simulink model "SubmarineFault"  (R2019a)
settings: Solver=ode1  StartTime=0.0  StopTime=2.5  FixedStep=Ts_Power  RelTol=1e-3
PostLoadFcn:
  | %% Init for wind PnO models - global system parameters
  | OVERRIDE_SSN_MEMORY_LIMIT=1;
  | Ts=50e-6;
  | % Ts=50e-10;
  | Ts_Power=Ts;
  | Ts_Control=2*Ts;
  | freq = 50;
  | Fnom=freq;
  | Vac=400e3;
InitFcn:
  | %% Init for wind PnO models - global system parameters
  | OVERRIDE_SSN_MEMORY_LIMIT=1;
  | Ts=50e-6;
  | % Ts=50e-10;
  | Ts_Power=Ts;
  | Ts_Control=2*Ts;
  | freq = 50;
  | Fnom=freq;
  | Vac=225e3;
values from neighbouring files (symbols this model uses):
  sub_posCap = 0.16e-006    (= 1.6e-07)    [variable.m]
  sub_posInd = 0.001400563    [variable.m]
  sub_posR = 0.036    [variable.m]
  sub_zeroCap = 0.053333e-006    (= 5.3333e-08)    [variable.m]
  sub_zeroInd = 0.00420169    [variable.m]
  sub_zeroR = 0.108    [variable.m]
  transfo_L1 = 0.05999374    [variable.m]
  transfo_L2 = 0.05999374    [variable.m]
  transfo_R1 = 0.000866667    [variable.m]
  transfo_R2 = 0.00086667    [variable.m]
undefined symbols (not defined in the file or in its folder): D1, D11, Delta, den, DiscIntNeverNeededParam, dx, find_system, gcbh, num, out_Buses, out_WindFarms, sps_rtmsupport
libraries: powerlib x168, simulink x80, powerlib_meascontrol x80, elements x52, eeSinusoidalMeasurement x46, simulink_extras x40, spsVIMeasurementModel x36, eePowerMeasurement x15
(part 6 of 22)

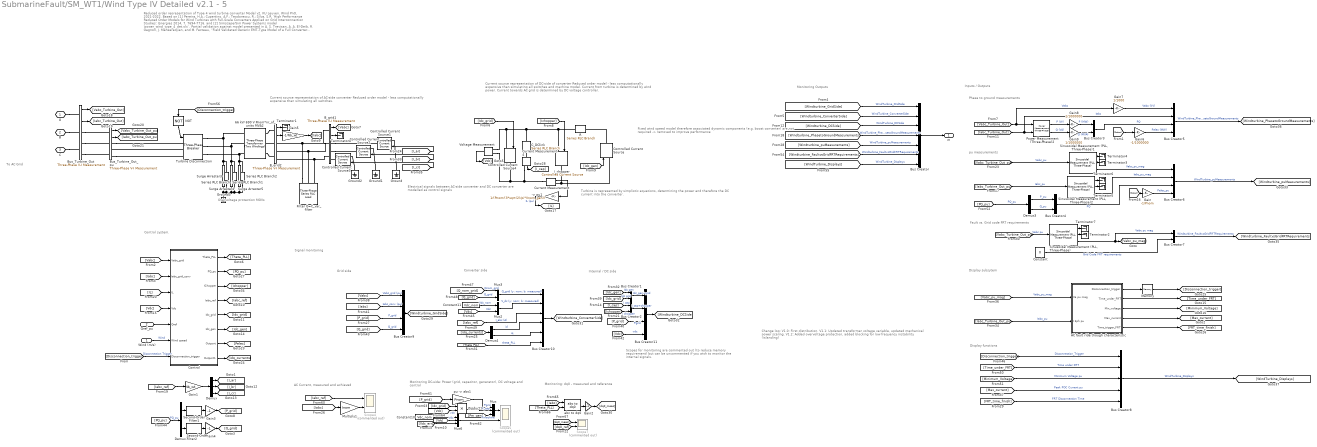
== system SubmarineFault/SM_WT1/Wind Type IV Detailed v2.1 - 5 ==
  note: Fault vs. Grid
      | code FRT
      | requirements
  note: pu measurements
  note: Control system.
  note: AC Current, measured and achieved
  note: Converter side
  note: Monitoring: dq0 - measured and reference
  note: Change log:
      | V1.0: First distribution.
      | V1.1: Updated transformer voltage variable, updated mechanical power scaling.
      | V1.2: Added overvoltage protection, added blocking for low frequency instability (islanding)
  note: Grid side
  note: Overvoltage
      | protection MOVs
  note: Internal / DC side
  note: Fixed wind speed model therefore associated dynamic components (e.g. boost converter) are not required -> removed to improve performance
  note: Scopes for monitoring are commented out (to reduce memory requirement) but can be uncommented if you wish to monitor the internal signals.
  note: Electrical signals between AC-side converter and DC converter are modelled as control signals
  note: Monitoring DC-side: Power (grid, capacitor, generator), DC voltage and control
  note: To AC Grid
  note: Monitoring Outputs
  note: Signal monitoring
  note: Current source representation of AC-side converter
      | Reduced order model - less computationally expensive than simulating all switches.
  note: Turbine is represented by simplistic equations, determining the power and therefore the DC current into the converter.
  note: Current source representation of DC-side of converter
      | Reduced order model - less computationally expensive than simulating all switches and machine model. Current from turbine is determined by wind power. Current towards AC grid is determined by DC voltage controller.
  note: Reduced order representation of Type 4 wind turbine converter
      | Model v2, KU Leuven, Wind PnO, 2021-2022.
      | Based on [1] Pereira, H.A.; Cupertino, A.F.; Teodorescu, R.; Silva, S.R. 'High Performance Reduced Order Models for Wind Turbines with Full-Scale Converters Applied on Grid Interconnection Studies'. Energies 2014, 7, 7694-7716. and [2] Simscape/Sim Power Systems model 'power_wind_type_4_det.slx' . Partial validation against model presented in A. S. Trevisan, A. A. El-Deib, R. Gagnon, J. Mahseredjian, and M. Fecteau, “Field Validated Generic EMT-Type Model of a Full Converter Wind Turbine Based on a Gearless Externally Excited Synchronous Generator,” IEEE Trans. Power Deliv., 2018. Developed with reduced complexity to allow for real time simulation in future sessions.
  note: Phase to ground measurements
  note: Display subsytem
  note: Display functions
  note: Inputs / Outputs
  "Wind (m/s) " : Inport
  Qref_pu : Inport  Port=2
  -> pu1 : Gain  Gain=1/(Pnom/(3*sqrt(2)/pi*Vnom_gen))  SaturateOnIntegerOverflow=on  OutDataTypeStr=Inherit: Same as input  ParamDataTypeStr=Inherit: Same as input
  66 kV/ 690 V Pnom*nr_of_units MVA2 : powerlib/Elements/Three-Phase Transformer (Two Windings)  Winding1Connection=Delta (D11)  Winding2Connection=Yg  CoreType=Three single-phase transformers  SetSaturation=off  Hysteresis=off  DataFile='hysteresis'  SetInitialFlux=off  Measurements=None  UNITS=pu  NominalPower="[Pnom*Nb_wt  freq]"  Winding1=[Vgrid 0.00083333 0.025]  Winding2=[690 0.00083333 0.025]  Rm=500  Lm=Inf  L0=0.5  Saturation=[0 0;0.0024 1.2;1 1.52]  InitialFluxes=[ 0.8 , -0.8 , 0.7 ]  BreakLoop=off  DiscreteSolver=Trapezoidal iterative  DataType=off  TransfoNumber=0
  AC fault ride though characteristic : Subsystem
  B_grid1 : powerlib/Measurements/Three-Phase V-I Measurement  VoltageMeasurement=phase-to-ground  SetLabelV=off  LabelV=Vabc  Vpu=on  VpuLL=off  CurrentMeasurement=yes  SetLabelI=off  LabelI=Iabc  Ipu=on  Pbase=Pnom  Vbase=Vnom  OutputType=Complex  PhasorSimulation=off  PSBequivalent=0
  B_grid2 : powerlib/Measurements/Three-Phase V-I Measurement  VoltageMeasurement=phase-to-ground  SetLabelV=off  LabelV=Vabc  Vpu=on  VpuLL=off  CurrentMeasurement=yes  SetLabelI=off  LabelI=Iabc  Ipu=on  Pbase=Pnom  Vbase=Vnom  OutputType=Complex  PhasorSimulation=off  PSBequivalent=0
  Bus Creator : BusCreator  Inputs=7
  Bus Creator{1..4,7} (5 alike) : BusCreator  Inputs=2
  Bus Creator10 : BusCreator  Inputs=6
  Bus Creator{5..6,9,11} (4 alike) : BusCreator  Inputs=4
  Bus Creator8 : BusCreator  Inputs=5
  Bus_Turbine_Out : powerlib/Measurements/Three-Phase V-I Measurement  VoltageMeasurement=phase-to-ground  SetLabelV=off  LabelV=Vabc_Turbine_Out  Vpu=off  VpuLL=off  CurrentMeasurement=yes  SetLabelI=off  LabelI=Iabc_Turbine_Out  Ipu=off  Pbase=Pnom  Vbase=Pnom  OutputType=Complex  PhasorSimulation=off  PSBequivalent=0
  Bus_Turbine_Out_pu : powerlib/Measurements/Three-Phase V-I Measurement  VoltageMeasurement=phase-to-phase  SetLabelV=off  LabelV=Vabc_Turbine_Out_pu  Vpu=off  VpuLL=on  CurrentMeasurement=yes  SetLabelI=off  LabelI=Iabc_Turbine_Out_pu  Ipu=on  Pbase=Pnom*Nb_wt  Vbase=Vgrid  OutputType=Complex  PhasorSimulation=off  PSBequivalent=0
  C_DClink : powerlib/Elements/Series RLC Branch  LConnTagsString=__new0  RConnTagsString=__new0  BranchType=C  Resistance=1  Inductance=1e-3  SetiL0=off  InitialCurrent=0  Capacitance=C_DClink  Setx0=on  InitialVoltage=Vdc_nom  Measurements=Branch voltage
  Constant : Constant  Value=0
  Constant10 : Constant  Value=Vdc_nom
  Constant11 : Constant  Value=Vdc_nom
  Control : Subsystem  mask{Freq=Freq_filter, Zeta=Zeta_filter, Ts=Ts}
      mask prompts: Freq "Cut-off frequency (Hz):"; Ts "Sample time"
  Controlled Current Source : powerlib/Electrical Sources/Controlled Current Source  Initialize=on  Source_Type=DC  Amplitude=0  Phase=0  Frequency=0  Measurements=None
  Controlled Current Source1 : powerlib/Electrical Sources/Controlled Current Source  Initialize=on  Source_Type=AC  Amplitude=0  Phase=0  Frequency=0  Measurements=None
  Controlled Current Source2 : powerlib/Electrical Sources/Controlled Current Source  Initialize=on  Source_Type=AC  Amplitude=0  Phase=0  Frequency=0  Measurements=None
  Controlled Current Source3 : powerlib/Electrical Sources/Controlled Current Source  Initialize=on  Source_Type=AC  Amplitude=0  Phase=0  Frequency=0  Measurements=None
  Controlled Current Source4 : powerlib/Electrical Sources/Controlled Current Source  Initialize=on  Source_Type=DC  Amplitude=0  Phase=0  Frequency=0  Measurements=None
  Current Measurement : powerlib/Measurements/Current Measurement  PhasorSimulation=off  OutputType=Complex  PSBequivalent=0
  Current Measurement4 : powerlib/Measurements/Current Measurement  PhasorSimulation=off  OutputType=Complex  PSBequivalent=0
  Demux : Demux  Outputs=3
  Demux1 : Demux  Outputs=2
  Demux3 : Demux  Outputs=2
  Demux4 : Demux  Outputs=2
  Filter Q=C_var_filter : powerlib/Elements/Three-Phase Series RLC Load  LConnTagsString=A|B|C  Configuration=Y (grounded)  NominalVoltage=Vnom  Vabc=[1e3 1e3 1e3]  Vabcp=[1e3 1e3 1e3]  NominalFrequency=freq  UnbalancedPower=off  ActivePower=Nb_wt*C_var_filter/Q_filter  InductivePower=0  CapacitivePower=Nb_wt*C_var_filter  Pabc=[10e3 9e3 11e3]  QLabc=[100 90 110]  QCabc=[100 90 110]  Pabcp=[10e3 9e3 11e3]  QLabcp=[100 90 110]  QCabcp=[100 90 110]  Measurements=None  LoadType=constant Z
  Gain : Gain  Gain=-1/Pnom
  Gain1 : Gain  Gain=Nb_wt
  Gain2 : Gain  Gain=-1
  Gain3 : Gain  Gain=-1
  Gain4 : Gain  Gain=-1
  Gain5 : Gain  Gain=-1/Nb_wt
  Gain6 : Gain  Gain=-1/1000000
  Gain7 : Gain  Gain=1/1000
  Gain8 : Gain  Gain=1/1000000
  Gain9 : Gain  Gain=1/1000000
  Ground{,1..3} (4 alike) : powerlib/Elements/Ground  LConnTagsString=a
  I_chopper : powerlib/Electrical Sources/Controlled Current Source  Initialize=on  Source_Type=AC  Amplitude=0  Phase=0  Frequency=0  Measurements=None
  Memory : Memory
  Multiply1 : Gain  Gain=Inom
  Mux : Mux  Inputs=3
  Mux2 : Mux  Inputs=2
  Mux3 : Mux  Inputs=2
  Mux6 : Mux  Inputs=3
  NOT : Logic  Operator=NOT  AllPortsSameDT=off  OutDataTypeStr=boolean
  Power Measurement (Three-Phase)2 : eePowerMeasurement/Power Measurement (Three-Phase)  LabelModeActiveChoice=Discrete  F=freq  K=1  Seq=Positive  Ts=Ts
      settings: SourceProductBaseCode=PS
  Product1 : Product
  R : powerlib/Elements/Series RLC Branch  LConnTagsString=__new0  RConnTagsString=__new0  BranchType=R  Resistance=0.01  Inductance=1e-3  SetiL0=off  InitialCurrent=0  Capacitance=C_DClink  Setx0=on  InitialVoltage=Vdc_nom  Measurements=Branch voltage
  Scope4 : Scope  Commented=on  NumInputPorts=2
  Scope5 : Scope  Commented=on  NumInputPorts=2
  Scope7 : Scope  Commented=on  NumInputPorts=2
  Second-Order Filter1 : powerlib_meascontrol/Filters/Second-Order Filter  FilterType=Lowpass  Fo=freq  Zeta=0.707  Ts=Ts  Initialize=off  Vac_Init="[0,  0,  60]"  Vdc_Init=0  PlotResponse=off  FreqRange=[0, 500, 1]
      settings: SourceProductBaseCode=PS
  Second-Order Filter2 : powerlib_meascontrol/Filters/Second-Order Filter  FilterType=Lowpass  Fo=freq  Zeta=0.707  Ts=Ts  Initialize=off  Vac_Init="[0,  0,  60]"  Vdc_Init=0  PlotResponse=off  FreqRange=[0, 500, 1]
      settings: SourceProductBaseCode=PS
  Series RLC Branch : powerlib/Elements/Series RLC Branch  LConnTagsString=__new0  RConnTagsString=__new0  BranchType=R  Resistance=1e9  Inductance=1e-3  SetiL0=off  InitialCurrent=0  Capacitance=1e-6  Setx0=off  InitialVoltage=0  Measurements=None
  Series RLC Branch1 : powerlib/Elements/Series RLC Branch  LConnTagsString=__new0  RConnTagsString=__new0  BranchType=R  Resistance=1e9  Inductance=1e-3  SetiL0=off  InitialCurrent=0  Capacitance=1e-6  Setx0=off  InitialVoltage=0  Measurements=None
  Series RLC Branch2 : powerlib/Elements/Series RLC Branch  LConnTagsString=__new0  RConnTagsString=__new0  BranchType=R  Resistance=1e9  Inductance=1e-3  SetiL0=off  InitialCurrent=0  Capacitance=1e-6  Setx0=off  InitialVoltage=0  Measurements=None
  "Sinusoidal Measurement (PLL, Three-Phase)" : eeSinusoidalMeasurement/Sinusoidal Measurement (PLL, Three-Phase)  Kp_LF=200  Ki_LF=2000  F0=freq  Theta0=0  Ts=-1
      settings: SourceProductBaseCode=PS
  "Sinusoidal Measurement (PLL, Three-Phase)1" : eeSinusoidalMeasurement/Sinusoidal Measurement (PLL, Three-Phase)  Kp_LF=200  Ki_LF=2000  F0=freq  Theta0=0  Ts=-1
      settings: SourceProductBaseCode=PS
  "Sinusoidal Measurement (PLL, Three-Phase)2" : eeSinusoidalMeasurement/Sinusoidal Measurement (PLL, Three-Phase)  Kp_LF=200  Ki_LF=2000  F0=freq  Theta0=0  Ts=-1
      settings: SourceProductBaseCode=PS
  Surge Arrester3 : powerlib/Elements/Surge Arrester  ProtectionVoltage=90e+03  Columns=2  ReferenceCurrent=500  Segment1=[.955 50]  Segment2=[1.0 25]  Segment3=[.9915 16.5]  Measurements=None  BreakLoop=off  UseDiscreteRobustSolver=on
      settings: SourceProductBaseCode=PS
  Surge Arrester4 : powerlib/Elements/Surge Arrester  ProtectionVoltage=90e+03  Columns=2  ReferenceCurrent=500  Segment1=[.955 50]  Segment2=[1.0 25]  Segment3=[.9915 16.5]  Measurements=None  BreakLoop=off  UseDiscreteRobustSolver=on
      settings: SourceProductBaseCode=PS
  Surge Arrester5 : powerlib/Elements/Surge Arrester  ProtectionVoltage=90e+03  Columns=2  ReferenceCurrent=500  Segment1=[.955 50]  Segment2=[1.0 25]  Segment3=[.9915 16.5]  Measurements=None  BreakLoop=off  UseDiscreteRobustSolver=on
      settings: SourceProductBaseCode=PS
  Terminator{1..8} (8 alike) : Terminator
  Turbine Disconnection : powerlib/Elements/Three-Phase Breaker  InitialState=closed  SwitchA=on  SwitchB=on  SwitchC=on  SwitchTimes="[1/60  5/60]"  External=on  BreakerResistance=0.01  SnubberResistance=1e6  SnubberCapacitance=inf  Measurements=None
  Voltage Measurement : powerlib/Measurements/Voltage Measurement  PhasorSimulation=off  OutputType=Complex  PSBequivalent=0
  abc to dq0 : powerlib_meascontrol/Transformations/abc to dq0  Alignment=90 degrees behind phase A axis
  "pu -> abs1" : Gain  Gain=Pnom
  A : PMIOPort  Tag=PMCPort  Side=Left
  B : PMIOPort  Tag=PMCPort  Port=2  Side=Left
  C : PMIOPort  Tag=PMCPort  Port=3  Side=Left
  m : Outport  VectorParamsAs1DForOutWhenUnconnected=on
  wires:
  Bus Creator5/1 -> [Windturbine_PhasetoGroundMeasurements]  "WindTurbine_PhasetoGroundMeasurements"
  Bus Creator8/1 -> [WindTurbine_Displays]  "WindTurbine_Displays"
  [Windturbine_ConverterSide] -> Bus Creator/2  "WindTurbine_ConverterSide"
  NOT/1 -> Turbine Disconnection/1
  [Disconnection_trigger] -> NOT/1
  Memory/1 -> [Disconnection_trigger]
  [Disconnection_trigger] -> Bus Creator8/1  "Disconnection_Trigger"
  [WindTurbine_Displays] -> Bus Creator/7  "WindTurbine_Displays"
  [Windturbine_FaultvsGridFRTRequirements] -> Bus Creator/6  "Windturbine_FaultvsGridFRTRequirements"
  [Windturbine_DCSide] -> Bus Creator/3  "WindTurbine_DCSide"
  [Windturbine_puMeasurements] -> Bus Creator/5  "WindTurbine_puMeasurements"
  [Windturbine_PhasetoGroundMeasurements] -> Bus Creator/4  "WindTurbine_PhasetoGroundMeasurements"
  [Windturbine_GridSide] -> Bus Creator/1  "WindTurbine_GridSide"
  Bus Creator/1 -> m/1
  Bus Creator7/1 -> [Windturbine_FaultvsGridFRTRequirements]  "Windturbine_FaultvsGridFRTRequirements"
  Bus Creator6/1 -> [Windturbine_puMeasurements]  "WindTurbine_puMeasurements"
  Bus Creator11/1 -> [Windturbine_DCSide]
  Bus Creator10/1 -> [Windturbine_ConverterSide]
  Bus Creator9/1 -> [Windturbine_GridSide]
  [FRT_time_finish] -> Bus Creator8/5  "FRT Disconnection Time"
  AC fault ride though characteristic/5(Time_trigger_FRT) -> [FRT_time_finish]
  Gain9/1 -> Bus Creator3/2  "Q (MVA)"
  Gain8/1 -> Bus Creator3/1  "P (MW)"
  Gain7/1 -> Bus Creator5/1  "Vabc (kV)"
  [Disconnection_trigger] -> Control/7(Disconnection_trigger)  "Disconnection Trigger"
  AC fault ride though characteristic/1(Disconnection_trigger) -> Memory/1
  [idq_currents] -> Demux4/1
  Control/8(Outport1) -> [idq_currents]
  Control/7(Outport) -> [Pelec]
  [PQ_pu] -> Demux3/1  "PQ_pu"
  Bus_Turbine_Out_pu/2 -> [Iabc_Turbine_Out_pu]
  Bus_Turbine_Out_pu/1 -> [Vabc_Turbine_Out_pu]
  Bus_Turbine_Out/2 -> [Iabc_Turbine_Out]
  Bus_Turbine_Out/1 -> [Vabc_Turbine_Out]
  Constant/1 -> Bus Creator7/2  "Grid Code FRT requirements"
  [Time_under_FRT] -> Bus Creator8/2  "Time under FRT"
  [Minimum_Voltage] -> Bus Creator8/3  "Minimum Voltage pu"
  [Max_current] -> Bus Creator8/4  "Peak POC Current pu"
  [Vabc_pu_mag] -> AC fault ride though characteristic/1(Va pu mag)  "Vabc_pu_mag"
  [Iabc_Turbine_Out_pu] -> AC fault ride though characteristic/2(I 3ph pu)  "Iabc_pu"
  [Vabc_Turbine_Out_pu] -> "Sinusoidal Measurement (PLL, Three-Phase)"/1  "Vabc pu"
  "Sinusoidal Measurement (PLL, Three-Phase)"/1 -> Terminator7/1
  "Sinusoidal Measurement (PLL, Three-Phase)"/3 -> Bus Creator7/1, [Vabc_pu_mag]  "Vabc pu mag"
  "Sinusoidal Measurement (PLL, Three-Phase)"/2 -> Terminator2/1
  AC fault ride though characteristic/3(Min_voltage) -> [Minimum_Voltage]
  AC fault ride though characteristic/2(Time_under_FRT) -> [Time_under_FRT]
  AC fault ride though characteristic/4(Max_current) -> [Max_current]
  Bus Creator4/1 -> Bus Creator6/3  "PQ"
  Demux3/2 -> Bus Creator4/2  "Q_pu"
  Demux3/1 -> Bus Creator4/1  "P_pu"
  [Vabc_Turbine_Out_pu] -> "Sinusoidal Measurement (PLL, Three-Phase)1"/1  "Vabc_pu"
  [Iabc_Turbine_Out_pu] -> "Sinusoidal Measurement (PLL, Three-Phase)2"/1  "Iabc_pu"
  "Sinusoidal Measurement (PLL, Three-Phase)2"/3 -> Bus Creator6/2  "Iabc_pu_mag"
  [Pelec] -> Gain/1
  "Sinusoidal Measurement (PLL, Three-Phase)1"/1 -> Terminator4/1
  Gain/1 -> Bus Creator6/4  "Pelec_pu"
  "Sinusoidal Measurement (PLL, Three-Phase)2"/2 -> Terminator5/1
  "Sinusoidal Measurement (PLL, Three-Phase)1"/3 -> Bus Creator6/1  "Vabc_pu_mag"
  "Sinusoidal Measurement (PLL, Three-Phase)1"/2 -> Terminator3/1
  "Sinusoidal Measurement (PLL, Three-Phase)2"/1 -> Terminator6/1
  [Iabc_Turbine_Out] -> Power Measurement (Three-Phase)2/2, Bus Creator5/2  "Iabc"
  Power Measurement (Three-Phase)2/1 -> Gain8/1  "P (W)"
  Gain6/1 -> Bus Creator5/4  "Pelec (MW)"
  [Vabc_Turbine_Out] -> Gain7/1, Power Measurement (Three-Phase)2/1  "Vabc"
  Bus Creator3/1 -> Bus Creator5/3  "PQ"
  Power Measurement (Three-Phase)2/2 -> Gain9/1  "Q (VA)"
  [Pelec] -> Gain6/1
  [I_cr] -> Controlled Current Source3/1
  Current Measurement/1 -> -> pu1/1
  [Ichopper] -> Bus Creator2/2  "I chopper"
  [Vdc] -> Control/4(Vdc)
  [Iabc_ref] -> Scope4/1
  Multiply1/1 -> Scope4/2
  -> pu1/1 -> [IL]  "IL (pu)"
  [Iabc] -> Control/2(Iabc_grid_conv)
  Qref_pu/1 -> Control/5(Qref)
  Demux/3 -> [I_cr]
  Mux2/1 -> Bus Creator10/2  "V_dc (y: nom; b: measured)"
  [Theta_PLL] -> abc to dq0/2
  [P_grid] -> Bus Creator9/3  "P_grid"
  [Iabc] -> abc to dq0/1
  Demux/2 -> [I_br]
  Demux4/2 -> Bus Creator10/5  "iq"
  [Vabc] -> Control/1(Vabc_grid)
  [Q_grid] -> Mux3/2  "Q_grid"
  Demux4/1 -> Bus Creator10/4  "id"
  [Vabc] -> Bus Creator9/1  "Vabc_grid (pu)"
  [Iabc] -> Bus Creator9/2  "Iabc_conv (pu)"
  [Q_nom_grid] -> Mux3/1  "Qnom_grid"
  [Theta_PLL] -> Bus Creator10/6  "theta_PLL"
  [IL] -> Control/3(IL)
  [Q_grid] -> Bus Creator9/4  "Q_grid"
  Mux3/1 -> Bus Creator10/1  "Q_grid (y: nom; b: measured)"
  Control/2(PQ_pu) -> [PQ_pu]
  Control/1(Theta_PLL) -> [Theta_PLL]
  [Iabc_ref] -> Bus Creator10/3  "I_abc (A)"
  abc to dq0/1 -> Gain2/1
  Voltage Measurement/1 -> [Vdc]
  Bus Creator1/1 -> Bus Creator11/1  "Idc_gen+grid"
  [I_cap] -> Bus Creator2/1  "I cap"
  [P_grid] -> "pu -> abs1"/1
  [I_ar] -> Controlled Current Source1/1
  [Pm_gen] -> Mux/3  "Pmachine"
  [Iabc] -> Multiply1/1
  [dq0_meas] -> Scope7/1
  [Vdc] -> Bus Creator11/4  "vdc"
  [P_grid] -> Bus Creator11/3  "Pgrid"
  [Idc_gen] -> Bus Creator1/1  "Idc gen"
  Demux1/2 -> Second-Order Filter2/1
  [Idc_grid] -> Bus Creator1/2  "Idc grid"
  Second-Order Filter2/1 -> Gain4/1
  Bus Creator2/1 -> Bus Creator11/2  "I_cap+chopper"
  Gain2/1 -> [dq0_meas]
  [Vdc_err] -> Mux6/3
  [Iabc_ref] -> Gain1/1
  Constant10/1 -> Mux6/1
  Control/3(IChopper) -> [Ichopper]
  Control/4(Iabc_ref) -> [Iabc_ref]
  Current Measurement4/1 -> [I_cap]
  [Idc_grid] -> Product1/1
  Constant11/1 -> Mux2/1  "Vdc_nom"
  B_grid1/1 -> [Vabc]
  [I_br] -> Controlled Current Source2/1
  Gain3/1 -> [P_grid]
  [Vdc] -> Mux2/2  "Vdc"
  [Idc_gen] -> Controlled Current Source/1
  Product1/1 -> Mux/2  "P_cap"
  Gain5/1 -> [Iabc]
  Control/6(Idc_gen) -> [Idc_gen]
  B_grid1/2 -> Terminator8/1
  [Vdc] -> Mux6/2  "Vdc"
  Second-Order Filter1/1 -> Gain3/1
  [Ichopper] -> I_chopper/1
  B_grid2/1 -> Terminator1/1
  [Vdc] -> Product1/2  "vdc"
  Gain1/1 -> Demux/1
  Mux6/1 -> Scope5/2
  [dq0_ref] -> Scope7/2
  Demux/1 -> [I_ar]
  Control/5(Idc_grid) -> [Idc_grid]
  Gain4/1 -> [Q_grid]
  Mux/1 -> Scope5/1
  "pu -> abs1"/1 -> Mux/1  "Pgrid"
  [PQ_pu] -> Demux1/1  "PQ_pu"
  Demux1/1 -> Second-Order Filter1/1
  [Idc_grid] -> Controlled Current Source4/1
  B_grid2/2 -> Gain5/1
  "Wind (m/s) "/1 -> Control/6(Wind speed)  "Wind"
  connections:
  Bus_Turbine_Out_pu/RConn3 -- Turbine Disconnection/LConn3
  Turbine Disconnection/LConn2 -- Bus_Turbine_Out_pu/RConn2
  Bus_Turbine_Out_pu/RConn1 -- Turbine Disconnection/LConn1
  Filter Q=C_var_filter/LConn1 -- B_grid2/RConn1 -- B_grid1/LConn1
  Bus_Turbine_Out/RConn3 -- Bus_Turbine_Out_pu/LConn3
  Bus_Turbine_Out/RConn2 -- Bus_Turbine_Out_pu/LConn2
  Bus_Turbine_Out/RConn1 -- Bus_Turbine_Out_pu/LConn1
  C/RConn1 -- Bus_Turbine_Out/LConn3
  B/RConn1 -- Bus_Turbine_Out/LConn2
  A/RConn1 -- Bus_Turbine_Out/LConn1
  Ground/LConn1 -- Controlled Current Source1/LConn1
  B_grid1/RConn3 -- Controlled Current Source3/RConn1
  Controlled Current Source/RConn1 -- R/LConn1
  Ground2/LConn1 -- Controlled Current Source3/LConn1
  Ground1/LConn1 -- Controlled Current Source2/LConn1
  B_grid1/RConn2 -- Controlled Current Source2/RConn1
  B_grid1/RConn1 -- Controlled Current Source1/RConn1
  B_grid2/LConn2 -- 66 kV/ 690 V Pnom*nr_of_units MVA2/RConn2
  B_grid2/LConn3 -- 66 kV/ 690 V Pnom*nr_of_units MVA2/RConn3
  Current Measurement4/LConn1 -- C_DClink/RConn1
  B_grid2/LConn1 -- 66 kV/ 690 V Pnom*nr_of_units MVA2/RConn1
  B_grid2/RConn3 -- Filter Q=C_var_filter/LConn3 -- B_grid1/LConn3
  Current Measurement/LConn1 -- Current Measurement4/RConn1 -- Voltage Measurement/LConn2 -- Controlled Current Source4/RConn1
  Controlled Current Source/LConn1 -- I_chopper/RConn1 -- Current Measurement/RConn1
  B_grid2/RConn2 -- Filter Q=C_var_filter/LConn2 -- B_grid1/LConn2
  Controlled Current Source4/LConn1 -- C_DClink/LConn1 -- R/RConn1 -- I_chopper/LConn1 -- Voltage Measurement/LConn1
  Turbine Disconnection/RConn3 -- 66 kV/ 690 V Pnom*nr_of_units MVA2/LConn3 -- Series RLC Branch2/LConn1 -- Surge Arrester5/LConn1
  Turbine Disconnection/RConn2 -- 66 kV/ 690 V Pnom*nr_of_units MVA2/LConn2 -- Surge Arrester4/LConn1 -- Series RLC Branch1/LConn1
  Turbine Disconnection/RConn1 -- 66 kV/ 690 V Pnom*nr_of_units MVA2/LConn1 -- Surge Arrester3/LConn1 -- Series RLC Branch/LConn1
  Surge Arrester5/RConn1 -- Series RLC Branch2/RConn1 -- Series RLC Branch1/RConn1 -- Surge Arrester3/RConn1 -- Ground3/LConn1 -- Series RLC Branch/RConn1 -- Surge Arrester4/RConn1

== system SubmarineFault/SM_WT1/Differential Element 1/Main Protection (Current Differential) ==
  IA : Inport
  IB : Inport  Port=2
  IC : Inport  Port=3
  VA : Inport  Port=4
  VB : Inport  Port=5
  VC : Inport  Port=6
  IAR : Inport  Port=7
  IBR : Inport  Port=8
  ICR : Inport  Port=9
  Charging Current Compensation phase A : Subsystem
  Charging Current Compensation phase B : Subsystem
  Charging Current Compensation phase C : Subsystem
  Current Differential Protection for Phase A : Subsystem
  Current Differential Protection for Phase B : Subsystem
  Current Differential Protection for Phase C : Subsystem
  Trip A : Outport  InitialOutput=0  VectorParamsAs1DForOutWhenUnconnected=on
  Trip B : Outport  Port=2  InitialOutput=0  VectorParamsAs1DForOutWhenUnconnected=on
  Trip C : Outport  Port=3  InitialOutput=0  VectorParamsAs1DForOutWhenUnconnected=on
  wires:
  VC/1 -> Charging Current Compensation phase B/3(VC), Charging Current Compensation phase C/3(VC), Charging Current Compensation phase A/3(VC)
  VB/1 -> Charging Current Compensation phase B/2(VB), Charging Current Compensation phase C/2(VB), Charging Current Compensation phase A/2(VB)
  Charging Current Compensation phase C/1(Icomp) -> Current Differential Protection for Phase C/3(Icomp)
  Charging Current Compensation phase B/1(Icomp) -> Current Differential Protection for Phase B/3(Icomp)
  Charging Current Compensation phase A/1(Icomp) -> Current Differential Protection for Phase A/3(Icomp)
  VA/1 -> Charging Current Compensation phase A/1(VA), Charging Current Compensation phase C/1(VA), Charging Current Compensation phase B/1(VA)
  ICR/1 -> Current Differential Protection for Phase C/2(Iremote)
  IC/1 -> Current Differential Protection for Phase C/1(Ilocal)
  IBR/1 -> Current Differential Protection for Phase B/2(Iremote)
  Current Differential Protection for Phase B/1(Trip) -> Trip B/1
  Current Differential Protection for Phase A/1(Trip) -> Trip A/1
  Current Differential Protection for Phase C/1(Trip) -> Trip C/1
  IB/1 -> Current Differential Protection for Phase B/1(Ilocal)
  IAR/1 -> Current Differential Protection for Phase A/2(Iremote)
  IA/1 -> Current Differential Protection for Phase A/1(Ilocal)

== system SubmarineFault/SM_WT1/Differential Element 2/Main Protection (Current Differential) ==
  IA : Inport
  IB : Inport  Port=2
  IC : Inport  Port=3
  VA : Inport  Port=4
  VB : Inport  Port=5
  VC : Inport  Port=6
  IAR : Inport  Port=7
  IBR : Inport  Port=8
  ICR : Inport  Port=9
  Charging Current Compensation phase A : Subsystem
  Charging Current Compensation phase B : Subsystem
  Charging Current Compensation phase C : Subsystem
  Current Differential Protection for Phase A : Subsystem
  Current Differential Protection for Phase B : Subsystem
  Current Differential Protection for Phase C : Subsystem
  Trip A : Outport  InitialOutput=0  VectorParamsAs1DForOutWhenUnconnected=on
  Trip B : Outport  Port=2  InitialOutput=0  VectorParamsAs1DForOutWhenUnconnected=on
  Trip C : Outport  Port=3  InitialOutput=0  VectorParamsAs1DForOutWhenUnconnected=on
  wires:
  VC/1 -> Charging Current Compensation phase B/3(VC), Charging Current Compensation phase C/3(VC), Charging Current Compensation phase A/3(VC)
  VB/1 -> Charging Current Compensation phase B/2(VB), Charging Current Compensation phase C/2(VB), Charging Current Compensation phase A/2(VB)
  Charging Current Compensation phase C/1(Icomp) -> Current Differential Protection for Phase C/3(Icomp)
  Charging Current Compensation phase B/1(Icomp) -> Current Differential Protection for Phase B/3(Icomp)
  Charging Current Compensation phase A/1(Icomp) -> Current Differential Protection for Phase A/3(Icomp)
  VA/1 -> Charging Current Compensation phase A/1(VA), Charging Current Compensation phase C/1(VA), Charging Current Compensation phase B/1(VA)
  ICR/1 -> Current Differential Protection for Phase C/2(Iremote)
  IC/1 -> Current Differential Protection for Phase C/1(Ilocal)
  IBR/1 -> Current Differential Protection for Phase B/2(Iremote)
  Current Differential Protection for Phase B/1(Trip) -> Trip B/1
  Current Differential Protection for Phase A/1(Trip) -> Trip A/1
  Current Differential Protection for Phase C/1(Trip) -> Trip C/1
  IB/1 -> Current Differential Protection for Phase B/1(Ilocal)
  IAR/1 -> Current Differential Protection for Phase A/2(Iremote)
  IA/1 -> Current Differential Protection for Phase A/1(Ilocal)

== system SubmarineFault/SM_WT1/Fault_timing_generator/faultgen ==
  t : Inport
  Tstat : Inport  Port=2
  Tdur : Inport  Port=3
  Add : Sum
  Logical Operator : Logic  AllPortsSameDT=off  OutDataTypeStr=boolean
  Relational Operator1 : RelationalOperator  Operator=<=  OutDataTypeStr=boolean  RndMeth=Nearest
  Relational Operatr : RelationalOperator  OutDataTypeStr=boolean  RndMeth=Nearest
  Scope : Scope  NumInputPorts=3
  fault : Outport  VectorParamsAs1DForOutWhenUnconnected=on
  wires:
  Add/1 -> Relational Operator1/2
  Relational Operator1/1 -> Scope/3, Logical Operator/2
  Relational Operatr/1 -> Logical Operator/1
  t/1 -> Scope/1, Relational Operatr/1, Relational Operator1/1
  Logical Operator/1 -> fault/1
  Tdur/1 -> Add/2
  Tstat/1 -> Scope/2, Relational Operatr/2, Add/1

== system SubmarineFault/SM_WT1/Fault_timing_generator/sawtooth ==
  Taqu : Inport
  pules : Inport  Port=2
  Constant : Constant
  Data Type Conversion : DataTypeConversion
  Discrete-Time Integrator : DiscreteIntegrator  ExternalReset=rising  SampleTime=-1  ICPrevOutput=DiscIntNeverNeededParam  ICPrevScaledInput=DiscIntNeverNeededParam
  Logical Operator : Logic  AllPortsSameDT=off
  Memory : Memory
  Relational Operator : RelationalOperator  OutDataTypeStr=boolean  RndMeth=Nearest
  sawtooth : Outport  VectorParamsAs1DForOutWhenUnconnected=on
  trig : Outport  Port=2  VectorParamsAs1DForOutWhenUnconnected=on
  wires:
  Constant/1 -> Discrete-Time Integrator/1
  Discrete-Time Integrator/1 -> Memory/1, sawtooth/1
  Memory/1 -> Relational Operator/1
  Logical Operator/1 -> Discrete-Time Integrator/2, Data Type Conversion/1
  Relational Operator/1 -> Logical Operator/2
  pules/1 -> Logical Operator/1
  Taqu/1 -> Relational Operator/2
  Data Type Conversion/1 -> trig/1

== system SubmarineFault/SM_WT1/Impedance Element 1/Impedance Relay Scheme ==
  note: Impedance Relay Scheme
  Vabc : Inport
  Iabc : Inport  Port=2
  " 7" : Product  RndMeth=Zero
  "Analog filtering, signal conditioning" : Subsystem
  Combination of Voltages and Currents into 6 pairs (for each type of fault) : Subsystem
  DFT delay : TransportDelay  DelayTime=0.017  BufferSize=30720
  Fault A-B-C Measurement : Subsystem
  Fault A-G Measurement : Subsystem
  Fault B-C Measurement : Subsystem
  Fault B-G Measurement : Subsystem
  Fault C-A Measurement : Subsystem
  Fault C-G Measurement : Subsystem
  Logic Matrix : Subsystem
  Mux{,1,3..6} (6 alike) : Mux
  Mux2 : Mux  Inputs=2
  Product : Product  RndMeth=Zero
  Step1 : Step  Time=0.017  SampleTime=0
  Tripping Logic : Subsystem
  Undervoltage : Subsystem
  tm1 : Terminator
  "TRIP " : Outport  InitialOutput=0  VectorParamsAs1DForOutWhenUnconnected=on
  Logic : Outport  Port=2  InitialOutput=0  VectorParamsAs1DForOutWhenUnconnected=on
  FaultType : Outport  Port=3  InitialOutput=0  VectorParamsAs1DForOutWhenUnconnected=on
  FaultZone : Outport  Port=4  InitialOutput=0  VectorParamsAs1DForOutWhenUnconnected=on
  wires:
  Mux2/1 -> tm1/1
  Tripping Logic/3(Fault Zone) -> FaultZone/1
  Product/1 -> Tripping Logic/5(<V), Fault A-B-C Measurement/2(<V), Fault C-A Measurement/2(<V), Fault B-C Measurement/2(<V), Fault C-G Measurement/2(<V), Fault B-G Measurement/2(<V), Fault A-G Measurement/2(<V)
  Logic Matrix/5(Fault Type) -> FaultType/1
  Tripping Logic/2(Logic Signals) -> Logic/1
  Tripping Logic/1(TRIP) -> "TRIP "/1
  Logic Matrix/4(" Zone4") -> Tripping Logic/4(zone4)
  Logic Matrix/3(" Zone3") -> Tripping Logic/3(zone3)
  Logic Matrix/2(" Zone2") -> Tripping Logic/2(zone2)
  Logic Matrix/1(" Zone1") -> Tripping Logic/1(zone1)
  Mux6/1 -> Logic Matrix/6(A-B-C)
  Mux5/1 -> Logic Matrix/5(C-A)
  Mux4/1 -> Logic Matrix/4(B-C)
  Mux3/1 -> Logic Matrix/3(C-G)
  Mux1/1 -> Logic Matrix/2(B-G)
  Mux/1 -> Logic Matrix/1(A-G)
  Fault A-B-C Measurement/4(Zone4) -> Mux6/4
  Fault A-B-C Measurement/3(Zone3) -> Mux6/3
  Fault A-B-C Measurement/2(Zone2) -> Mux6/2
  Fault A-B-C Measurement/1(Zone1) -> Mux6/1
  Fault C-A Measurement/4(Zone4) -> Mux5/4
  Fault C-A Measurement/3(Zone3) -> Mux5/3
  Fault C-A Measurement/2(Zone2) -> Mux5/2
  Fault C-A Measurement/1(Zone1) -> Mux5/1
  Fault B-C Measurement/4(Zone4) -> Mux4/4
  Fault B-C Measurement/3(Zone3) -> Mux4/3
  Fault B-C Measurement/2(Zone2) -> Mux4/2
  Fault B-C Measurement/1(Zone1) -> Mux4/1
  Fault C-G Measurement/4(Zone4) -> Mux3/4
  Fault C-G Measurement/3(Zone3) -> Mux3/3
  Fault C-G Measurement/2(Zone2) -> Mux3/2
  Fault C-G Measurement/1(Zone1) -> Mux3/1
  Fault B-G Measurement/4(Zone4) -> Mux1/4
  Fault B-G Measurement/3(Zone3) -> Mux1/3
  Fault B-G Measurement/2(Zone2) -> Mux1/2
  Fault B-G Measurement/1(Zone1) -> Mux1/1
  Fault A-G Measurement/4(Zone4) -> Mux/4
  Fault A-G Measurement/3(Zone3) -> Mux/3
  Fault A-G Measurement/2(Zone2) -> Mux/2
  Fault A-G Measurement/1(Zone1) -> Mux/1
  DFT delay/1 -> Product/1
  Combination of Voltages and Currents into 6 pairs (for each type of fault)/6("Volt, Curr A-B,A-B-C-G") -> Fault A-B-C Measurement/1(A-B-C)
  Combination of Voltages and Currents into 6 pairs (for each type of fault)/5("Volt, Curr C-A,C-A-G") -> Fault C-A Measurement/1(C-A)
  Combination of Voltages and Currents into 6 pairs (for each type of fault)/4("Volt, Curr B-C,B-C-G") -> Fault B-C Measurement/1(B-C)
  Combination of Voltages and Currents into 6 pairs (for each type of fault)/3("Volt, Curr C-G") -> Fault C-G Measurement/1(C-G)
  Combination of Voltages and Currents into 6 pairs (for each type of fault)/2("Volt, Curr B-G") -> Fault B-G Measurement/1(B-G)
  "Analog filtering, signal conditioning"/3(If0) -> Combination of Voltages and Currents into 6 pairs (for each type of fault)/3(If0)
  "Analog filtering, signal conditioning"/2(If) -> Combination of Voltages and Currents into 6 pairs (for each type of fault)/2(If)
  "Analog filtering, signal conditioning"/5(if) -> Mux2/2
  "Analog filtering, signal conditioning"/4(vf) -> Mux2/1
  "Analog filtering, signal conditioning"/1(Vf) -> Undervoltage/1("Vabc  "), Combination of Voltages and Currents into 6 pairs (for each type of fault)/1(Vf)
  " 7"/1 -> Product/2, DFT delay/1
  Step1/1 -> " 7"/2
  Undervoltage/1(<V) -> " 7"/1
  Combination of Voltages and Currents into 6 pairs (for each type of fault)/1("Volt, Curr A-G") -> Fault A-G Measurement/1(A-G)
  Iabc/1 -> "Analog filtering, signal conditioning"/2(Iin)
  Vabc/1 -> "Analog filtering, signal conditioning"/1(Vin)

== system SubmarineFault/SM_WT1/Impedance Element 2/Impedance Relay Scheme ==
  note: Impedance Relay Scheme
  Vabc : Inport
  Iabc : Inport  Port=2
  " 7" : Product  RndMeth=Zero
  "Analog filtering, signal conditioning" : Subsystem
  Combination of Voltages and Currents into 6 pairs (for each type of fault) : Subsystem
  DFT delay : TransportDelay  DelayTime=0.017  BufferSize=30720
  Fault A-B-C Measurement : Subsystem
  Fault A-G Measurement : Subsystem
  Fault B-C Measurement : Subsystem
  Fault B-G Measurement : Subsystem
  Fault C-A Measurement : Subsystem
  Fault C-G Measurement : Subsystem
  Logic Matrix : Subsystem
  Mux{,1,3..6} (6 alike) : Mux
  Mux2 : Mux  Inputs=2
  Product : Product  RndMeth=Zero
  Step1 : Step  Time=0.017  SampleTime=0
  Tripping Logic : Subsystem
  Undervoltage : Subsystem
  tm1 : Terminator
  "TRIP " : Outport  InitialOutput=0  VectorParamsAs1DForOutWhenUnconnected=on
  Logic : Outport  Port=2  InitialOutput=0  VectorParamsAs1DForOutWhenUnconnected=on
  FaultType : Outport  Port=3  InitialOutput=0  VectorParamsAs1DForOutWhenUnconnected=on
  FaultZone : Outport  Port=4  InitialOutput=0  VectorParamsAs1DForOutWhenUnconnected=on
  wires:
  Mux2/1 -> tm1/1
  Tripping Logic/3(Fault Zone) -> FaultZone/1
  Product/1 -> Tripping Logic/5(<V), Fault A-B-C Measurement/2(<V), Fault C-A Measurement/2(<V), Fault B-C Measurement/2(<V), Fault C-G Measurement/2(<V), Fault B-G Measurement/2(<V), Fault A-G Measurement/2(<V)
  Logic Matrix/5(Fault Type) -> FaultType/1
  Tripping Logic/2(Logic Signals) -> Logic/1
  Tripping Logic/1(TRIP) -> "TRIP "/1
  Logic Matrix/4(" Zone4") -> Tripping Logic/4(zone4)
  Logic Matrix/3(" Zone3") -> Tripping Logic/3(zone3)
  Logic Matrix/2(" Zone2") -> Tripping Logic/2(zone2)
  Logic Matrix/1(" Zone1") -> Tripping Logic/1(zone1)
  Mux6/1 -> Logic Matrix/6(A-B-C)
  Mux5/1 -> Logic Matrix/5(C-A)
  Mux4/1 -> Logic Matrix/4(B-C)
  Mux3/1 -> Logic Matrix/3(C-G)
  Mux1/1 -> Logic Matrix/2(B-G)
  Mux/1 -> Logic Matrix/1(A-G)
  Fault A-B-C Measurement/4(Zone4) -> Mux6/4
  Fault A-B-C Measurement/3(Zone3) -> Mux6/3
  Fault A-B-C Measurement/2(Zone2) -> Mux6/2
  Fault A-B-C Measurement/1(Zone1) -> Mux6/1
  Fault C-A Measurement/4(Zone4) -> Mux5/4
  Fault C-A Measurement/3(Zone3) -> Mux5/3
  Fault C-A Measurement/2(Zone2) -> Mux5/2
  Fault C-A Measurement/1(Zone1) -> Mux5/1
  Fault B-C Measurement/4(Zone4) -> Mux4/4
  Fault B-C Measurement/3(Zone3) -> Mux4/3
  Fault B-C Measurement/2(Zone2) -> Mux4/2
  Fault B-C Measurement/1(Zone1) -> Mux4/1
  Fault C-G Measurement/4(Zone4) -> Mux3/4
  Fault C-G Measurement/3(Zone3) -> Mux3/3
  Fault C-G Measurement/2(Zone2) -> Mux3/2
  Fault C-G Measurement/1(Zone1) -> Mux3/1
  Fault B-G Measurement/4(Zone4) -> Mux1/4
  Fault B-G Measurement/3(Zone3) -> Mux1/3
  Fault B-G Measurement/2(Zone2) -> Mux1/2
  Fault B-G Measurement/1(Zone1) -> Mux1/1
  Fault A-G Measurement/4(Zone4) -> Mux/4
  Fault A-G Measurement/3(Zone3) -> Mux/3
  Fault A-G Measurement/2(Zone2) -> Mux/2
  Fault A-G Measurement/1(Zone1) -> Mux/1
  DFT delay/1 -> Product/1
  Combination of Voltages and Currents into 6 pairs (for each type of fault)/6("Volt, Curr A-B,A-B-C-G") -> Fault A-B-C Measurement/1(A-B-C)
  Combination of Voltages and Currents into 6 pairs (for each type of fault)/5("Volt, Curr C-A,C-A-G") -> Fault C-A Measurement/1(C-A)
  Combination of Voltages and Currents into 6 pairs (for each type of fault)/4("Volt, Curr B-C,B-C-G") -> Fault B-C Measurement/1(B-C)
  Combination of Voltages and Currents into 6 pairs (for each type of fault)/3("Volt, Curr C-G") -> Fault C-G Measurement/1(C-G)
  Combination of Voltages and Currents into 6 pairs (for each type of fault)/2("Volt, Curr B-G") -> Fault B-G Measurement/1(B-G)
  "Analog filtering, signal conditioning"/3(If0) -> Combination of Voltages and Currents into 6 pairs (for each type of fault)/3(If0)
  "Analog filtering, signal conditioning"/2(If) -> Combination of Voltages and Currents into 6 pairs (for each type of fault)/2(If)
  "Analog filtering, signal conditioning"/5(if) -> Mux2/2
  "Analog filtering, signal conditioning"/4(vf) -> Mux2/1
  "Analog filtering, signal conditioning"/1(Vf) -> Undervoltage/1("Vabc  "), Combination of Voltages and Currents into 6 pairs (for each type of fault)/1(Vf)
  " 7"/1 -> Product/2, DFT delay/1
  Step1/1 -> " 7"/2
  Undervoltage/1(<V) -> " 7"/1
  Combination of Voltages and Currents into 6 pairs (for each type of fault)/1("Volt, Curr A-G") -> Fault A-G Measurement/1(A-G)
  Iabc/1 -> "Analog filtering, signal conditioning"/2(Iin)
  Vabc/1 -> "Analog filtering, signal conditioning"/1(Vin)

== system SubmarineFault/SM_WT1/Overcurrent Element 1/Overcurrent Relay Scheme ==
  note: Overcurrent Relay Scheme
  Iabc : Inport
  "Analog filtering, signal conditioning" : Subsystem
  Data Type Conversion : DataTypeConversion  OutDataTypeStr=double
  Demux : Demux  Outputs=3
  Logic Matrix : Subsystem
  Phase A : Subsystem
  Phase B : Subsystem
  Phase C : Subsystem
  Residual : Subsystem
  Scope : Scope
  Tripping Logic : Subsystem
  tm1 : Terminator
  "TRIP " : Outport  InitialOutput=0  VectorParamsAs1DForOutWhenUnconnected=on
  Logic : Outport  Port=2  InitialOutput=0  VectorParamsAs1DForOutWhenUnconnected=on
  FaultType : Outport  Port=3  InitialOutput=0  VectorParamsAs1DForOutWhenUnconnected=on
  wires:
  Iabc/1 -> "Analog filtering, signal conditioning"/1(Iin)
  Tripping Logic/1(TRIP) -> "TRIP "/1
  Tripping Logic/2(Logic Signals) -> Logic/1
  "Analog filtering, signal conditioning"/1(If) -> Scope/1, Demux/1
  Demux/1 -> Phase A/1(IA)
  "Analog filtering, signal conditioning"/2(If0) -> Residual/1(IR)
  Demux/2 -> Phase B/1(IB)
  Demux/3 -> Phase C/1(IC)
  Phase A/1(Pickup) -> Logic Matrix/1(A)
  Phase B/1(Pickup) -> Logic Matrix/2(B)
  Phase C/1(Pickup) -> Logic Matrix/3(C)
  Residual/1(Pickup) -> Logic Matrix/4(R), Data Type Conversion/1
  Logic Matrix/1(" Op") -> Tripping Logic/1(Op)
  Logic Matrix/2(Fault Type) -> FaultType/1
  "Analog filtering, signal conditioning"/3(if) -> tm1/1
  Data Type Conversion/1 -> Tripping Logic/2(IR)

== system SubmarineFault/SM_WT1/Overcurrent Element 2/Overcurrent Relay Scheme ==
  note: Overcurrent Relay Scheme
  Iabc : Inport
  "Analog filtering, signal conditioning" : Subsystem
  Data Type Conversion : DataTypeConversion  OutDataTypeStr=double
  Demux : Demux  Outputs=3
  Logic Matrix : Subsystem
  Phase A : Subsystem
  Phase B : Subsystem
  Phase C : Subsystem
  Residual : Subsystem
  Tripping Logic : Subsystem
  tm1 : Terminator
  "TRIP " : Outport  InitialOutput=0  VectorParamsAs1DForOutWhenUnconnected=on
  Logic : Outport  Port=2  InitialOutput=0  VectorParamsAs1DForOutWhenUnconnected=on
  FaultType : Outport  Port=3  InitialOutput=0  VectorParamsAs1DForOutWhenUnconnected=on
  wires:
  Iabc/1 -> "Analog filtering, signal conditioning"/1(Iin)
  Tripping Logic/1(TRIP) -> "TRIP "/1
  Tripping Logic/2(Logic Signals) -> Logic/1
  "Analog filtering, signal conditioning"/1(If) -> Demux/1
  Demux/1 -> Phase A/1(IA)
  "Analog filtering, signal conditioning"/2(If0) -> Residual/1(IR)
  Demux/2 -> Phase B/1(IB)
  Demux/3 -> Phase C/1(IC)
  Phase A/1(Pickup) -> Logic Matrix/1(A)
  Phase B/1(Pickup) -> Logic Matrix/2(B)
  Phase C/1(Pickup) -> Logic Matrix/3(C)
  Residual/1(Pickup) -> Logic Matrix/4(R), Data Type Conversion/1
  Logic Matrix/1(" Op") -> Tripping Logic/1(Op)
  Logic Matrix/2(Fault Type) -> FaultType/1
  "Analog filtering, signal conditioning"/3(if) -> tm1/1
  Data Type Conversion/1 -> Tripping Logic/2(IR)

== system SubmarineFault/SM_WT1/Overcurrent Inverse time/Overcurrent Relay Scheme ==
  note: Overcurrent Relay Scheme
  Iabc : Inport
  "Analog filtering, signal conditioning" : Subsystem
  Demux : Demux  Outputs=3
  Logic Matrix : Subsystem
  Phase A : Subsystem
  Phase B : Subsystem
  Phase C : Subsystem
  Tripping Logic : Subsystem
  tm1 : Terminator
  tm2 : Terminator
  "TRIP " : Outport  InitialOutput=0  VectorParamsAs1DForOutWhenUnconnected=on
  FaultType : Outport  Port=2  InitialOutput=0  VectorParamsAs1DForOutWhenUnconnected=on
  wires:
  Tripping Logic/1(TRIP) -> "TRIP "/1
  "Analog filtering, signal conditioning"/1(If) -> Demux/1
  Demux/1 -> Phase A/1(IA)
  Demux/2 -> Phase B/1(IB)
  Demux/3 -> Phase C/1(IC)
  Phase A/1(Pickup) -> Logic Matrix/1(A)
  Phase B/1(Pickup) -> Logic Matrix/2(B)
  Phase C/1(Pickup) -> Logic Matrix/3(C)
  Logic Matrix/1(" Op") -> Tripping Logic/1(Op)
  Logic Matrix/2(Fault Type) -> FaultType/1
  "Analog filtering, signal conditioning"/3(if) -> tm1/1
  "Analog filtering, signal conditioning"/2(If0) -> tm2/1
  Iabc/1 -> "Analog filtering, signal conditioning"/1(Iin)

== system SubmarineFault/SM_WT1/Subsystem1/Subsystem ==
  V : Inport
  I : Inport  Port=2
  Bus Creator : BusCreator  Inputs=2
  Gain : Gain  Gain=1/1e6
  Gain1 : Gain  Gain=1/1e6
  Gain2 : Gain  Gain=1/1e3
  Gain3 : Gain  Gain=1/1e3
  Power Measurement (Three-Phase) : eePowerMeasurement/Power Measurement (Three-Phase)  LabelModeActiveChoice=Discrete  F=freq  K=1  Seq=Positive  Ts=Ts
      settings: SourceProductBaseCode=PS
  "Sinusoidal Measurement (PLL, Three-Phase)1" : eeSinusoidalMeasurement/Sinusoidal Measurement (PLL, Three-Phase)  Kp_LF=200  Ki_LF=2000  F0=freq  Theta0=0  Ts=-1
      settings: SourceProductBaseCode=PS
  "Sinusoidal Measurement (PLL, Three-Phase)6" : eeSinusoidalMeasurement/Sinusoidal Measurement (PLL, Three-Phase)  Kp_LF=200  Ki_LF=2000  F0=freq  Theta0=0  Ts=-1
      settings: SourceProductBaseCode=PS
  Terminator{,1..3} (4 alike) : Terminator
  Vabc : Outport  VectorParamsAs1DForOutWhenUnconnected=on
  Iabc : Outport  Port=2  VectorParamsAs1DForOutWhenUnconnected=on
  V mag : Outport  Port=3  VectorParamsAs1DForOutWhenUnconnected=on
  I mag : Outport  Port=4  VectorParamsAs1DForOutWhenUnconnected=on
  PQ : Outport  Port=5  VectorParamsAs1DForOutWhenUnconnected=on
  wires:
  Gain3/1 -> V mag/1  "V (kV)"
  I/1 -> Iabc/1, "Sinusoidal Measurement (PLL, Three-Phase)1"/1, Power Measurement (Three-Phase)/2  "I (A)"
  Power Measurement (Three-Phase)/1 -> Gain/1  "P (W)"
  Gain/1 -> Bus Creator/1  "P (MW)"
  Power Measurement (Three-Phase)/2 -> Gain1/1  "Q (VAr)"
  Bus Creator/1 -> PQ/1  "PQ"
  Gain1/1 -> Bus Creator/2  "Q (MVAr)"
  Gain2/1 -> Vabc/1  "V (kV)"
  V/1 -> Power Measurement (Three-Phase)/1, Gain2/1, "Sinusoidal Measurement (PLL, Three-Phase)6"/1  "V (V)"
  "Sinusoidal Measurement (PLL, Three-Phase)6"/2 -> Terminator/1
  "Sinusoidal Measurement (PLL, Three-Phase)6"/1 -> Terminator1/1
  "Sinusoidal Measurement (PLL, Three-Phase)6"/3 -> Gain3/1
  "Sinusoidal Measurement (PLL, Three-Phase)1"/3 -> I mag/1
  "Sinusoidal Measurement (PLL, Three-Phase)1"/1 -> Terminator3/1
  "Sinusoidal Measurement (PLL, Three-Phase)1"/2 -> Terminator2/1

== system SubmarineFault/SM_WT1/Subsystem10/Subsystem ==
  V : Inport
  I : Inport  Port=2
  Bus Creator : BusCreator  Inputs=2
  Gain : Gain  Gain=1/1e6
  Gain1 : Gain  Gain=1/1e6
  Gain2 : Gain  Gain=1/1e3
  Gain3 : Gain  Gain=1/1e3
  Power Measurement (Three-Phase) : eePowerMeasurement/Power Measurement (Three-Phase)  LabelModeActiveChoice=Discrete  F=freq  K=1  Seq=Positive  Ts=Ts
      settings: SourceProductBaseCode=PS
  "Sinusoidal Measurement (PLL, Three-Phase)1" : eeSinusoidalMeasurement/Sinusoidal Measurement (PLL, Three-Phase)  Kp_LF=200  Ki_LF=2000  F0=freq  Theta0=0  Ts=-1
      settings: SourceProductBaseCode=PS
  "Sinusoidal Measurement (PLL, Three-Phase)6" : eeSinusoidalMeasurement/Sinusoidal Measurement (PLL, Three-Phase)  Kp_LF=200  Ki_LF=2000  F0=freq  Theta0=0  Ts=-1
      settings: SourceProductBaseCode=PS
  Terminator{,1..3} (4 alike) : Terminator
  Vabc : Outport  VectorParamsAs1DForOutWhenUnconnected=on
  Iabc : Outport  Port=2  VectorParamsAs1DForOutWhenUnconnected=on
  V mag : Outport  Port=3  VectorParamsAs1DForOutWhenUnconnected=on
  I mag : Outport  Port=4  VectorParamsAs1DForOutWhenUnconnected=on
  PQ : Outport  Port=5  VectorParamsAs1DForOutWhenUnconnected=on
  wires:
  "Sinusoidal Measurement (PLL, Three-Phase)1"/2 -> Terminator2/1
  "Sinusoidal Measurement (PLL, Three-Phase)1"/1 -> Terminator3/1
  "Sinusoidal Measurement (PLL, Three-Phase)1"/3 -> I mag/1
  "Sinusoidal Measurement (PLL, Three-Phase)6"/3 -> Gain3/1
  "Sinusoidal Measurement (PLL, Three-Phase)6"/1 -> Terminator1/1
  "Sinusoidal Measurement (PLL, Three-Phase)6"/2 -> Terminator/1
  V/1 -> "Sinusoidal Measurement (PLL, Three-Phase)6"/1, Gain2/1, Power Measurement (Three-Phase)/1  "V (V)"
  Gain2/1 -> Vabc/1  "V (kV)"
  Gain1/1 -> Bus Creator/2  "Q (MVAr)"
  Bus Creator/1 -> PQ/1  "PQ"
  Power Measurement (Three-Phase)/2 -> Gain1/1  "Q (VAr)"
  Gain/1 -> Bus Creator/1  "P (MW)"
  Power Measurement (Three-Phase)/1 -> Gain/1  "P (W)"
  I/1 -> Power Measurement (Three-Phase)/2, "Sinusoidal Measurement (PLL, Three-Phase)1"/1, Iabc/1  "I (A)"
  Gain3/1 -> V mag/1  "V (kV)"

== system SubmarineFault/SM_WT1/Subsystem2/Subsystem ==
  V : Inport
  I : Inport  Port=2
  Bus Creator : BusCreator  Inputs=2
  Gain : Gain  Gain=1/1e6
  Gain1 : Gain  Gain=1/1e6
  Gain2 : Gain  Gain=1/1e3
  Gain3 : Gain  Gain=1/1e3
  Power Measurement (Three-Phase) : eePowerMeasurement/Power Measurement (Three-Phase)  LabelModeActiveChoice=Discrete  F=freq  K=1  Seq=Positive  Ts=Ts
      settings: SourceProductBaseCode=PS
  "Sinusoidal Measurement (PLL, Three-Phase)1" : eeSinusoidalMeasurement/Sinusoidal Measurement (PLL, Three-Phase)  Kp_LF=200  Ki_LF=2000  F0=freq  Theta0=0  Ts=-1
      settings: SourceProductBaseCode=PS
  "Sinusoidal Measurement (PLL, Three-Phase)6" : eeSinusoidalMeasurement/Sinusoidal Measurement (PLL, Three-Phase)  Kp_LF=200  Ki_LF=2000  F0=freq  Theta0=0  Ts=-1
      settings: SourceProductBaseCode=PS
  Terminator{,1..3} (4 alike) : Terminator
  Vabc : Outport  VectorParamsAs1DForOutWhenUnconnected=on
  Iabc : Outport  Port=2  VectorParamsAs1DForOutWhenUnconnected=on
  V mag : Outport  Port=3  VectorParamsAs1DForOutWhenUnconnected=on
  I mag : Outport  Port=4  VectorParamsAs1DForOutWhenUnconnected=on
  PQ : Outport  Port=5  VectorParamsAs1DForOutWhenUnconnected=on
  wires:
  "Sinusoidal Measurement (PLL, Three-Phase)1"/2 -> Terminator2/1
  "Sinusoidal Measurement (PLL, Three-Phase)1"/1 -> Terminator3/1
  "Sinusoidal Measurement (PLL, Three-Phase)1"/3 -> I mag/1
  "Sinusoidal Measurement (PLL, Three-Phase)6"/3 -> Gain3/1
  "Sinusoidal Measurement (PLL, Three-Phase)6"/1 -> Terminator1/1
  "Sinusoidal Measurement (PLL, Three-Phase)6"/2 -> Terminator/1
  V/1 -> "Sinusoidal Measurement (PLL, Three-Phase)6"/1, Gain2/1, Power Measurement (Three-Phase)/1  "V (V)"
  Gain2/1 -> Vabc/1  "V (kV)"
  Gain1/1 -> Bus Creator/2  "Q (MVAr)"
  Bus Creator/1 -> PQ/1  "PQ"
  Power Measurement (Three-Phase)/2 -> Gain1/1  "Q (VAr)"
  Gain/1 -> Bus Creator/1  "P (MW)"
  Power Measurement (Three-Phase)/1 -> Gain/1  "P (W)"
  I/1 -> Power Measurement (Three-Phase)/2, "Sinusoidal Measurement (PLL, Three-Phase)1"/1, Iabc/1  "I (A)"
  Gain3/1 -> V mag/1  "V (kV)"
